simulink model "someUnit"  (R2016b)
settings: Solver=VariableStepAuto  StartTime=0.0  StopTime=10.0  RelTol=1e-3
settings Model: Creator=zhoutinglin  LastModifiedBy=zhoutinglin

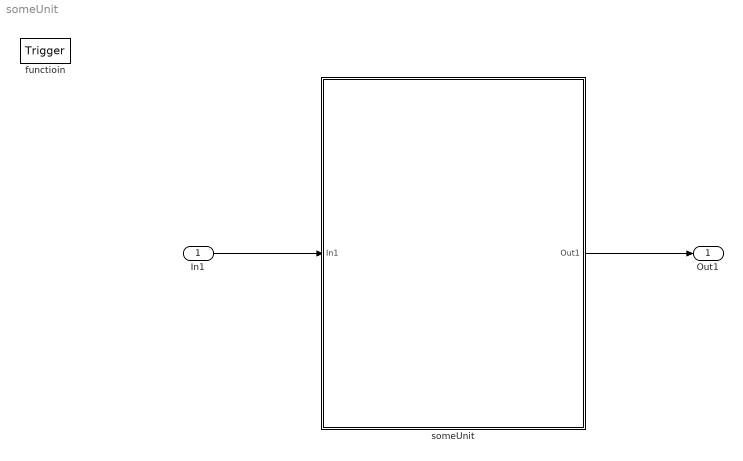
== system someUnit ==
  In1 : Inport
  functioin : TriggerPort  TriggerType=function-call  VariantControl=Variant  PortDimensions=1
  someUnit : Subsystem
  Out1 : Outport
  wires:
  In1/1 -> someUnit/1(In1)
  someUnit/1(Out1) -> Out1/1

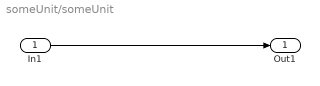
== system someUnit/someUnit ==
  In1 : Inport
  Out1 : Outport
  wires:
  In1/1 -> Out1/1
